simulink model "Ex2_5"  (R2016b)
settings: Solver=ode45  StartTime=0.0  StopTime=4  MaxStep=1e-3  RelTol=2e-3
values from neighbouring files (symbols this model uses):
  J1 = 10    [Ex2_5_init.m]
  J2 = 1    [Ex2_5_init.m]
  k = 100    [Ex2_2_init.m]    (also in Ex2_5_init.m = 5000)
  Tbrake = 50    [Ex2_5_init.m]
  w1_0 = 4    [Ex2_5_init.m]
  w2_0 = 4    [Ex2_5_init.m]
settings Model: Creator=Niels  LastModifiedBy=Niels

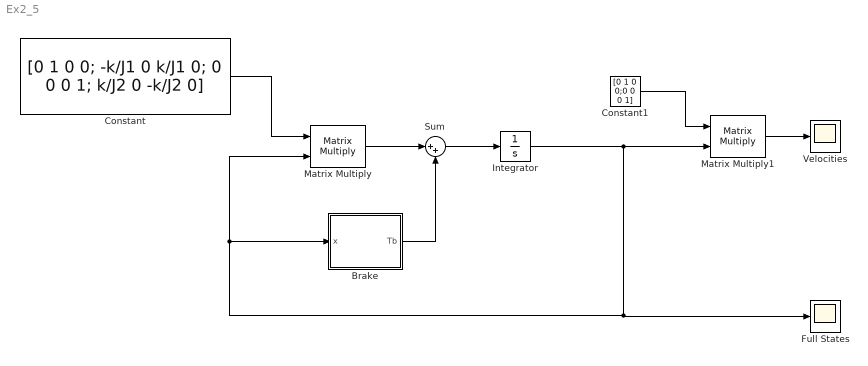
== system Ex2_5 ==
  Brake : MATLAB Function  TreatAsAtomicUnit=on
  Constant : Constant  Value=[0 1 0 0; -k/J1 0 k/J1 0; 0 0 0 1; k/J2 0 -k/J2 0]
  Constant1 : Constant  Value=[0 1 0 0;0 0 0 1]
  Full States : Scope
  Integrator : Integrator  InitialCondition=[0;w1_0;0;w2_0]
  Matrix Multiply : Product  Multiplication=Matrix(*)
  Matrix Multiply1 : Product  Multiplication=Matrix(*)
  Sum : Sum  Inputs=|++
  "Velocities " : Scope
  wires:
  Matrix Multiply/1 -> Sum/1
  Sum/1 -> Integrator/1
  Integrator/1 -> Matrix Multiply1/2, Full States/1, Matrix Multiply/2, Brake/1(x)
  Constant/1 -> Matrix Multiply/1
  Brake/1(Tb) -> Sum/2
  Matrix Multiply1/1 -> "Velocities "/1
  Constant1/1 -> Matrix Multiply1/1

== matlab function Ex2_5/Brake ==
  data: x input; Tb output; Tbrake parameter; J2 parameter; k parameter
function Tb = fcn(x,Tbrake, J2,k)
w2 = x(4); 
Tb = zeros(4,1);
T2 = abs(k*(x(1)-x(3)));
if w2 > 0.001
    Tb(4) = -Tbrake/J2;
elseif w2 < 0.001 
    Tb(4) = Tbrake/J2;
else
    Tb(4) = -sign(T2)*min(Tbrake,abs(T2) );
end
